simulink model "FOC_PMSM_FVSensorNew_testing"  (R2018b)
settings: Solver=ode45  StartTime=0  StopTime=0.2  FixedStep=1/fs/4  MaxStep=1/fs/2  RelTol=1e-7  EnableMultiTasking=on
InitFcn:
  | Motor_parameters_Lsrpm7fw
values from neighbouring files (symbols this model uses):
  fs = 20e3    (= 20000)    [Motor_parameters_Lsrpm7fw.m]
  Iphmax = I_rated*sqrt(2)*3    [Motor_parameters_Lsrpm7fw.m]
  J = 1*1e-3    (= 0.001)    [Motor_parameters_Lsrpm7fw.m]
  Ki1 = 2    [Motor_parameters_Lsrpm7fw.m]
  Ki2 = 6000    [Motor_parameters_Lsrpm7fw.m]
  Ki_pll = Bw^2*(1.1-0.334*zeta)^2*1/(2*k1)    (= 426432.888597)    [Motor_parameters_Lsrpm7fw.m]
  Kp1 = 0.05    [Motor_parameters_Lsrpm7fw.m]
  Kp2 = 6    [Motor_parameters_Lsrpm7fw.m]
  Kp_pll = Bw*(2.2*zeta-0.668*zeta^2)*1/(2*k1)    (= 13960.00992)    [Motor_parameters_Lsrpm7fw.m]
  Ld = 10e-3    (= 0.01)    [Motor_parameters_Lsrpm7fw.m]
  Lndd_ini = Lndmpm    (= 0.412)    [Motor_parameters_Lsrpm7fw.m]
  Lndmpm = 0.412    [Motor_parameters_Lsrpm7fw.m]
  Lq = 12.8e-3    (= 0.0128)    [Motor_parameters_Lsrpm7fw.m]
  Npp = 8/2    (= 4)    [Motor_parameters_Lsrpm7fw.m]
  Omegae_ini = 0    [Motor_parameters_Lsrpm7fw.m]
  Rs = 0.78    [Motor_parameters_Lsrpm7fw.m]
  Tl_const = Trat/nrat^2    (= 1.24081632653e-05)    [Motor_parameters_Lsrpm7fw.m]
  Trat = 38    [Motor_parameters_Lsrpm7fw.m]
  Vm = 70    [Motor_parameters_Lsrpm7fw.m]
  Vph = Vs*sqrt(2)    [Motor_parameters_Lsrpm7fw.m]
undefined symbols (not defined in the file or in its folder): DiscIntNeverNeededParam, plecs, sigbuilder_block
libraries: simulink x1
(part 2 of 2)

== system FOC_PMSM_FVSensorNew_testing/Rotor Pos. estimation/Cal. stator flux linkage/MinMax detection ==
  In : Inport
  Gain : Gain  Gain=1/2
  Max. Det : Subsystem
  Min. Det : Subsystem
  Mux6 : Mux  Inputs=3
  Scope5 : Scope
  Sum : Sum  Inputs=|++
  max.ou : Outport
  min.ou : Outport  Port=2
  average : Outport  Port=3
  wires:
  Gain/1 -> average/1
  Sum/1 -> Gain/1
  Max. Det/1(Max) -> max.ou/1, Mux6/1, Sum/1
  Min. Det/1(Min) -> min.ou/1, Mux6/3, Sum/2
  Mux6/1 -> Scope5/1
  In/1 -> Max. Det/1(In), Min. Det/1(In), Mux6/2

== system FOC_PMSM_FVSensorNew_testing/Rotor Pos. estimation/Cal. stator flux linkage1/MinMax detection ==
  In : Inport
  Gain : Gain  Gain=1/2
  Max. Det : Subsystem
  Min. Det : Subsystem
  Mux6 : Mux  Inputs=3
  Scope5 : Scope
  Sum : Sum  Inputs=|++
  max.ou : Outport
  min.ou : Outport  Port=2
  average : Outport  Port=3
  wires:
  Gain/1 -> average/1
  Sum/1 -> Gain/1
  Max. Det/1(Max) -> max.ou/1, Mux6/1, Sum/1
  Min. Det/1(Min) -> min.ou/1, Mux6/3, Sum/2
  Mux6/1 -> Scope5/1
  In/1 -> Max. Det/1(In), Min. Det/1(In), Mux6/2

== system FOC_PMSM_FVSensorNew_testing/Switch logic for sensorless vs sensor mode/Scope/ InputMux  ==
  In1 : Inport
  Convert1 : DataTypeConversion  SaturateOnIntegerOverflow=on  RndMeth=Zero
  Mux : Mux  Inputs=1
  Out : Outport
  wires:
  Convert1/1 -> Mux/1
  In1/1 -> Convert1/1
  Mux/1 -> Out/1

== system FOC_PMSM_FVSensorNew_testing/Switch logic for sensorless vs sensor mode/Scope1/ InputMux  ==
  In1 : Inport
  Convert1 : DataTypeConversion  SaturateOnIntegerOverflow=on  RndMeth=Zero
  Mux : Mux  Inputs=1
  Out : Outport
  wires:
  Mux/1 -> Out/1
  In1/1 -> Convert1/1
  Convert1/1 -> Mux/1

== system FOC_PMSM_FVSensorNew_testing/Rotor Pos. estimation/Cal. stator flux linkage/MinMax detection/Max. Det ==
  In : Inport
  Counter.1 : Subsystem
  Counter.2 : Subsystem
  Gain1 : Gain
  Gain2 : Gain  Gain=0.3
  Gain3 : Gain  Gain=0.6
  Mux2 : Mux
  Product : Product  RndMeth=Zero
  Relational Operator : RelationalOperator  RndMeth=Nearest
  Scope3 : Scope
  Unit Delay : UnitDelay  SampleTime=-1
  max.1 : Subsystem
  max.3 : Subsystem
  Max : Outport
  wires:
  Unit Delay/1 -> Relational Operator/2
  In/1 -> Unit Delay/1, max.1/1(In), Relational Operator/1, Mux2/1
  Relational Operator/1 -> max.1/Trigger, Counter.1/1(Sig.In), Counter.2/1(Sig.In), Gain1/1
  max.1/1(Out) -> max.3/1(In)
  Counter.1/1(En) -> Product/2, Gain3/1
  Mux2/1 -> Scope3/1
  Counter.2/1(En) -> Product/1, Gain2/1
  Product/1 -> max.3/Trigger
  Gain1/1 -> Mux2/2
  Gain2/1 -> Mux2/3
  Gain3/1 -> Mux2/4
  max.3/1(Out) -> Max/1

== system FOC_PMSM_FVSensorNew_testing/Rotor Pos. estimation/Cal. stator flux linkage/MinMax detection/Min. Det ==
  In : Inport
  Counter.1 : Subsystem
  Counter.2 : Subsystem
  Gain1 : Gain
  Gain2 : Gain  Gain=0.3
  Gain3 : Gain  Gain=0.6
  Mux2 : Mux
  Product : Product  RndMeth=Zero
  Relational Operator : RelationalOperator  Operator=<=  RndMeth=Nearest
  Scope3 : Scope
  Unit Delay : UnitDelay  SampleTime=-1
  max.1 : Subsystem
  max.3 : Subsystem
  Min : Outport
  wires:
  max.3/1(Out) -> Min/1
  Gain3/1 -> Mux2/4
  Gain2/1 -> Mux2/3
  Gain1/1 -> Mux2/2
  Product/1 -> max.3/Trigger
  Counter.2/1(En) -> Gain2/1, Product/1
  Mux2/1 -> Scope3/1
  Counter.1/1(En) -> Gain3/1, Product/2
  max.1/1(Out) -> max.3/1(In)
  Relational Operator/1 -> Gain1/1, Counter.2/1(Sig.In), Counter.1/1(Sig.In), max.1/Trigger
  In/1 -> Mux2/1, Relational Operator/1, max.1/1(In), Unit Delay/1
  Unit Delay/1 -> Relational Operator/2

== system FOC_PMSM_FVSensorNew_testing/Rotor Pos. estimation/Cal. stator flux linkage1/MinMax detection/Max. Det ==
  In : Inport
  Counter.1 : Subsystem
  Counter.2 : Subsystem
  Gain1 : Gain
  Gain2 : Gain  Gain=0.3
  Gain3 : Gain  Gain=0.6
  Mux2 : Mux
  Product : Product  RndMeth=Zero
  Relational Operator : RelationalOperator  RndMeth=Nearest
  Scope3 : Scope
  Unit Delay : UnitDelay  SampleTime=-1
  max.1 : Subsystem
  max.3 : Subsystem
  Max : Outport
  wires:
  Unit Delay/1 -> Relational Operator/2
  In/1 -> Unit Delay/1, max.1/1(In), Relational Operator/1, Mux2/1
  Relational Operator/1 -> max.1/Trigger, Counter.1/1(Sig.In), Counter.2/1(Sig.In), Gain1/1
  max.1/1(Out) -> max.3/1(In)
  Counter.1/1(En) -> Product/2, Gain3/1
  Mux2/1 -> Scope3/1
  Counter.2/1(En) -> Product/1, Gain2/1
  Product/1 -> max.3/Trigger
  Gain1/1 -> Mux2/2
  Gain2/1 -> Mux2/3
  Gain3/1 -> Mux2/4
  max.3/1(Out) -> Max/1

== system FOC_PMSM_FVSensorNew_testing/Rotor Pos. estimation/Cal. stator flux linkage1/MinMax detection/Min. Det ==
  In : Inport
  Counter.1 : Subsystem
  Counter.2 : Subsystem
  Gain1 : Gain
  Gain2 : Gain  Gain=0.3
  Gain3 : Gain  Gain=0.6
  Mux2 : Mux
  Product : Product  RndMeth=Zero
  Relational Operator : RelationalOperator  Operator=<=  RndMeth=Nearest
  Scope3 : Scope
  Unit Delay : UnitDelay  SampleTime=-1
  max.1 : Subsystem
  max.3 : Subsystem
  Min : Outport
  wires:
  max.3/1(Out) -> Min/1
  Gain3/1 -> Mux2/4
  Gain2/1 -> Mux2/3
  Gain1/1 -> Mux2/2
  Product/1 -> max.3/Trigger
  Counter.2/1(En) -> Gain2/1, Product/1
  Mux2/1 -> Scope3/1
  Counter.1/1(En) -> Gain3/1, Product/2
  max.1/1(Out) -> max.3/1(In)
  Relational Operator/1 -> Gain1/1, Counter.2/1(Sig.In), Counter.1/1(Sig.In), max.1/Trigger
  In/1 -> Mux2/1, Relational Operator/1, max.1/1(In), Unit Delay/1
  Unit Delay/1 -> Relational Operator/2

== system FOC_PMSM_FVSensorNew_testing/Rotor Pos. estimation/Cal. stator flux linkage/MinMax detection/Max. Det/Counter.1 ==
  Sig.In : Inport
  Constant4 : Constant  Value=10
  Constant5 : Constant
  Conter with enable : Subsystem
  Sum1 : Sum  Inputs=|-+
  En : Outport
  wires:
  Constant5/1 -> Sum1/2
  Sig.In/1 -> Sum1/1
  Conter with enable/1(Max. Reached?) -> En/1
  Sum1/1 -> Conter with enable/1(_|  |_)
  Constant4/1 -> Conter with enable/2(Max. Num)

== system FOC_PMSM_FVSensorNew_testing/Rotor Pos. estimation/Cal. stator flux linkage/MinMax detection/Max. Det/Counter.2 ==
  Sig.In : Inport
  Constant4 : Constant  Value=5
  Conter with enable : Subsystem
  Gain : Gain  Gain=2
  Gain1 : Gain  Gain=3
  Gain2 : Gain  Gain=4
  Mux1 : Mux
  Rising edge gen. : Subsystem
  SR Latch : Subsystem
  Scope2 : Scope
  En : Outport
  wires:
  Constant4/1 -> Conter with enable/2(Max. Num)
  Sig.In/1 -> Conter with enable/1(_|  |_), Rising edge gen./1(_|  |_), Gain2/1
  Conter with enable/1(Max. Reached?) -> SR Latch/2(S), Gain1/1
  SR Latch/1(Q) -> En/1, Mux1/1
  Mux1/1 -> Scope2/1
  Rising edge gen./1(Edge) -> SR Latch/1(R), Gain/1
  Gain/1 -> Mux1/2
  Gain1/1 -> Mux1/3
  Gain2/1 -> Mux1/4

== system FOC_PMSM_FVSensorNew_testing/Rotor Pos. estimation/Cal. stator flux linkage/MinMax detection/Max. Det/max.1 ==
  In : Inport
  Trigger : TriggerPort  TriggerType=falling  VariantControl=(inherit)
  Out : Outport
  wires:
  In/1 -> Out/1

== system FOC_PMSM_FVSensorNew_testing/Rotor Pos. estimation/Cal. stator flux linkage/MinMax detection/Max. Det/max.3 ==
  In : Inport
  Trigger : TriggerPort  VariantControl=(inherit)
  Out : Outport
  wires:
  In/1 -> Out/1

== system FOC_PMSM_FVSensorNew_testing/Rotor Pos. estimation/Cal. stator flux linkage/MinMax detection/Min. Det/Counter.1 ==
  Sig.In : Inport
  Constant4 : Constant  Value=10
  Constant5 : Constant
  Conter with enable : Subsystem
  Sum1 : Sum  Inputs=|-+
  En : Outport
  wires:
  Constant4/1 -> Conter with enable/2(Max. Num)
  Sum1/1 -> Conter with enable/1(_|  |_)
  Conter with enable/1(Max. Reached?) -> En/1
  Sig.In/1 -> Sum1/1
  Constant5/1 -> Sum1/2

== system FOC_PMSM_FVSensorNew_testing/Rotor Pos. estimation/Cal. stator flux linkage/MinMax detection/Min. Det/Counter.2 ==
  Sig.In : Inport
  Constant4 : Constant  Value=5
  Conter with enable : Subsystem
  Gain : Gain  Gain=2
  Gain1 : Gain  Gain=3
  Gain2 : Gain  Gain=4
  Mux1 : Mux
  Rising edge gen. : Subsystem
  SR Latch : Subsystem
  Scope2 : Scope
  En : Outport
  wires:
  Gain2/1 -> Mux1/4
  Gain1/1 -> Mux1/3
  Gain/1 -> Mux1/2
  Rising edge gen./1(Edge) -> Gain/1, SR Latch/1(R)
  Mux1/1 -> Scope2/1
  SR Latch/1(Q) -> Mux1/1, En/1
  Conter with enable/1(Max. Reached?) -> Gain1/1, SR Latch/2(S)
  Sig.In/1 -> Gain2/1, Rising edge gen./1(_|  |_), Conter with enable/1(_|  |_)
  Constant4/1 -> Conter with enable/2(Max. Num)

== system FOC_PMSM_FVSensorNew_testing/Rotor Pos. estimation/Cal. stator flux linkage/MinMax detection/Min. Det/max.1 ==
  In : Inport
  Trigger : TriggerPort  TriggerType=falling  VariantControl=(inherit)
  Out : Outport
  wires:
  In/1 -> Out/1

== system FOC_PMSM_FVSensorNew_testing/Rotor Pos. estimation/Cal. stator flux linkage/MinMax detection/Min. Det/max.3 ==
  In : Inport
  Trigger : TriggerPort  VariantControl=(inherit)
  Out : Outport
  wires:
  In/1 -> Out/1

== system FOC_PMSM_FVSensorNew_testing/Rotor Pos. estimation/Cal. stator flux linkage1/MinMax detection/Max. Det/Counter.1 ==
  Sig.In : Inport
  Constant4 : Constant  Value=10
  Constant5 : Constant
  Conter with enable : Subsystem
  Sum1 : Sum  Inputs=|-+
  En : Outport
  wires:
  Constant5/1 -> Sum1/2
  Sig.In/1 -> Sum1/1
  Conter with enable/1(Max. Reached?) -> En/1
  Sum1/1 -> Conter with enable/1(_|  |_)
  Constant4/1 -> Conter with enable/2(Max. Num)

== system FOC_PMSM_FVSensorNew_testing/Rotor Pos. estimation/Cal. stator flux linkage1/MinMax detection/Max. Det/Counter.2 ==
  Sig.In : Inport
  Constant4 : Constant  Value=5
  Conter with enable : Subsystem
  Gain : Gain  Gain=2
  Gain1 : Gain  Gain=3
  Gain2 : Gain  Gain=4
  Mux1 : Mux
  Rising edge gen. : Subsystem
  SR Latch : Subsystem
  Scope2 : Scope
  En : Outport
  wires:
  Constant4/1 -> Conter with enable/2(Max. Num)
  Sig.In/1 -> Conter with enable/1(_|  |_), Rising edge gen./1(_|  |_), Gain2/1
  Conter with enable/1(Max. Reached?) -> SR Latch/2(S), Gain1/1
  SR Latch/1(Q) -> En/1, Mux1/1
  Mux1/1 -> Scope2/1
  Rising edge gen./1(Edge) -> SR Latch/1(R), Gain/1
  Gain/1 -> Mux1/2
  Gain1/1 -> Mux1/3
  Gain2/1 -> Mux1/4

== system FOC_PMSM_FVSensorNew_testing/Rotor Pos. estimation/Cal. stator flux linkage1/MinMax detection/Max. Det/max.1 ==
  In : Inport
  Trigger : TriggerPort  TriggerType=falling  VariantControl=(inherit)
  Out : Outport
  wires:
  In/1 -> Out/1

== system FOC_PMSM_FVSensorNew_testing/Rotor Pos. estimation/Cal. stator flux linkage1/MinMax detection/Max. Det/max.3 ==
  In : Inport
  Trigger : TriggerPort  VariantControl=(inherit)
  Out : Outport
  wires:
  In/1 -> Out/1

== system FOC_PMSM_FVSensorNew_testing/Rotor Pos. estimation/Cal. stator flux linkage1/MinMax detection/Min. Det/Counter.1 ==
  Sig.In : Inport
  Constant4 : Constant  Value=10
  Constant5 : Constant
  Conter with enable : Subsystem
  Sum1 : Sum  Inputs=|-+
  En : Outport
  wires:
  Constant4/1 -> Conter with enable/2(Max. Num)
  Sum1/1 -> Conter with enable/1(_|  |_)
  Conter with enable/1(Max. Reached?) -> En/1
  Sig.In/1 -> Sum1/1
  Constant5/1 -> Sum1/2

== system FOC_PMSM_FVSensorNew_testing/Rotor Pos. estimation/Cal. stator flux linkage1/MinMax detection/Min. Det/Counter.2 ==
  Sig.In : Inport
  Constant4 : Constant  Value=5
  Conter with enable : Subsystem
  Gain : Gain  Gain=2
  Gain1 : Gain  Gain=3
  Gain2 : Gain  Gain=4
  Mux1 : Mux
  Rising edge gen. : Subsystem
  SR Latch : Subsystem
  Scope2 : Scope
  En : Outport
  wires:
  Gain2/1 -> Mux1/4
  Gain1/1 -> Mux1/3
  Gain/1 -> Mux1/2
  Rising edge gen./1(Edge) -> Gain/1, SR Latch/1(R)
  Mux1/1 -> Scope2/1
  SR Latch/1(Q) -> Mux1/1, En/1
  Conter with enable/1(Max. Reached?) -> Gain1/1, SR Latch/2(S)
  Sig.In/1 -> Gain2/1, Rising edge gen./1(_|  |_), Conter with enable/1(_|  |_)
  Constant4/1 -> Conter with enable/2(Max. Num)

== system FOC_PMSM_FVSensorNew_testing/Rotor Pos. estimation/Cal. stator flux linkage1/MinMax detection/Min. Det/max.1 ==
  In : Inport
  Trigger : TriggerPort  TriggerType=falling  VariantControl=(inherit)
  Out : Outport
  wires:
  In/1 -> Out/1

== system FOC_PMSM_FVSensorNew_testing/Rotor Pos. estimation/Cal. stator flux linkage1/MinMax detection/Min. Det/max.3 ==
  In : Inport
  Trigger : TriggerPort  VariantControl=(inherit)
  Out : Outport
  wires:
  In/1 -> Out/1

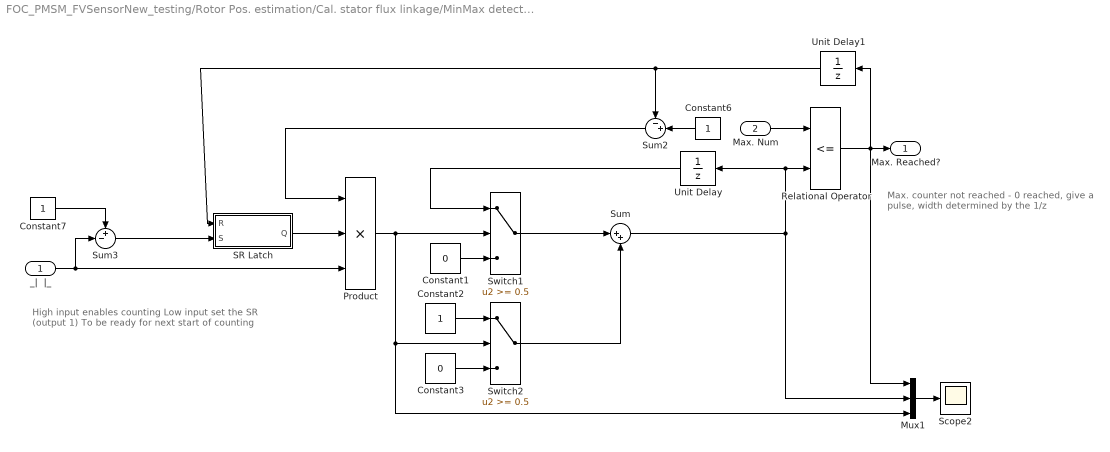
== system FOC_PMSM_FVSensorNew_testing/Rotor Pos. estimation/Cal. stator flux linkage/MinMax detection/Max. Det/Counter.1/Conter with enable ==
  note: High input enables counting
      | Low input set the SR (output 1)
      | To be ready for next start of
      | counting
  note: Max. counter not reached - 0
      | reached, give a pulse, width
      | determined by the 1/z
  _|  |_ : Inport
  Max. Num : Inport  Port=2
  Constant1 : Constant  Value=0
  Constant2 : Constant
  Constant3 : Constant  Value=0
  Constant6 : Constant
  Constant7 : Constant
  Mux1 : Mux  Inputs=3
  Product : Product  Inputs=3  RndMeth=Zero
  Relational Operator : RelationalOperator  Operator=<=  RndMeth=Nearest
  SR Latch : Subsystem
  Scope2 : Scope
  Sum : Sum  Inputs=|++
  Sum2 : Sum  Inputs=-+|
  Sum3 : Sum  Inputs=+-|
  Switch1 : Switch  Threshold=0.5
  Switch2 : Switch  Threshold=0.5
  Unit Delay : UnitDelay  SampleTime=-1
  Unit Delay1 : UnitDelay  SampleTime=-1
  Max. Reached? : Outport
  wires:
  Constant1/1 -> Switch1/3
  Constant2/1 -> Switch2/1
  Constant3/1 -> Switch2/3
  Switch1/1 -> Sum/1
  Switch2/1 -> Sum/2
  Sum/1 -> Unit Delay/1, Relational Operator/2, Mux1/2
  Unit Delay/1 -> Switch1/1
  Max. Num/1 -> Relational Operator/1
  Relational Operator/1 -> Mux1/1, Unit Delay1/1, Max. Reached?/1
  Mux1/1 -> Scope2/1
  Sum2/1 -> Product/1
  Product/1 -> Switch1/2, Switch2/2, Mux1/3
  _|  |_/1 -> Sum3/2, Product/3
  SR Latch/1(Q) -> Product/2
  Sum3/1 -> SR Latch/2(S)
  Constant7/1 -> Sum3/1
  Constant6/1 -> Sum2/2
  Unit Delay1/1 -> Sum2/1, SR Latch/1(R)

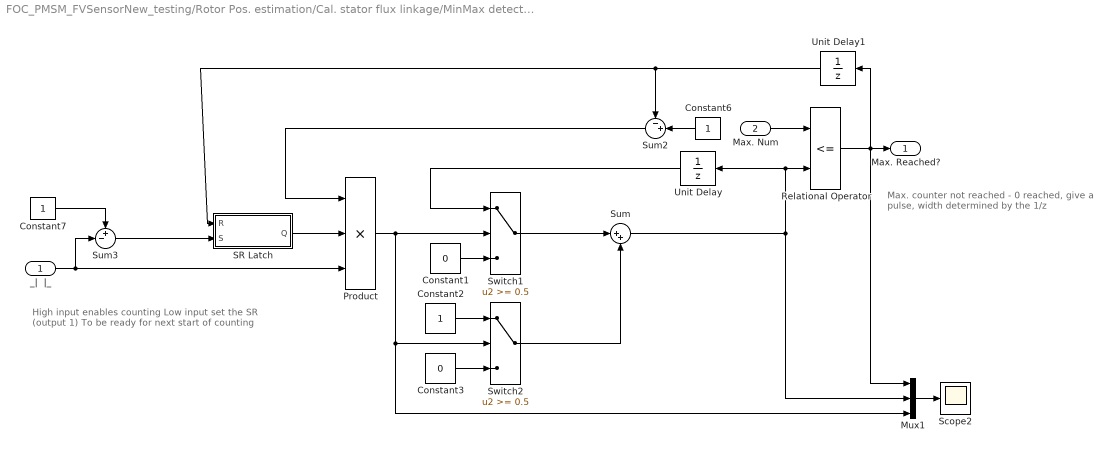
== system FOC_PMSM_FVSensorNew_testing/Rotor Pos. estimation/Cal. stator flux linkage/MinMax detection/Max. Det/Counter.2/Conter with enable ==
  note: Max. counter not reached - 0
      | reached, give a pulse, width
      | determined by the 1/z
  note: High input enables counting
      | Low input set the SR (output 1)
      | To be ready for next start of
      | counting
  _|  |_ : Inport
  Max. Num : Inport  Port=2
  Constant1 : Constant  Value=0
  Constant2 : Constant
  Constant3 : Constant  Value=0
  Constant6 : Constant
  Constant7 : Constant
  Mux1 : Mux  Inputs=3
  Product : Product  Inputs=3  RndMeth=Zero
  Relational Operator : RelationalOperator  Operator=<=  RndMeth=Nearest
  SR Latch : Subsystem
  Scope2 : Scope
  Sum : Sum  Inputs=|++
  Sum2 : Sum  Inputs=-+|
  Sum3 : Sum  Inputs=+-|
  Switch1 : Switch  Threshold=0.5
  Switch2 : Switch  Threshold=0.5
  Unit Delay : UnitDelay  SampleTime=-1
  Unit Delay1 : UnitDelay  SampleTime=-1
  Max. Reached? : Outport
  wires:
  Unit Delay1/1 -> SR Latch/1(R), Sum2/1
  Constant6/1 -> Sum2/2
  Constant7/1 -> Sum3/1
  Sum3/1 -> SR Latch/2(S)
  SR Latch/1(Q) -> Product/2
  _|  |_/1 -> Product/3, Sum3/2
  Product/1 -> Mux1/3, Switch2/2, Switch1/2
  Sum2/1 -> Product/1
  Mux1/1 -> Scope2/1
  Relational Operator/1 -> Max. Reached?/1, Unit Delay1/1, Mux1/1
  Max. Num/1 -> Relational Operator/1
  Unit Delay/1 -> Switch1/1
  Sum/1 -> Mux1/2, Relational Operator/2, Unit Delay/1
  Switch2/1 -> Sum/2
  Switch1/1 -> Sum/1
  Constant3/1 -> Switch2/3
  Constant2/1 -> Switch2/1
  Constant1/1 -> Switch1/3

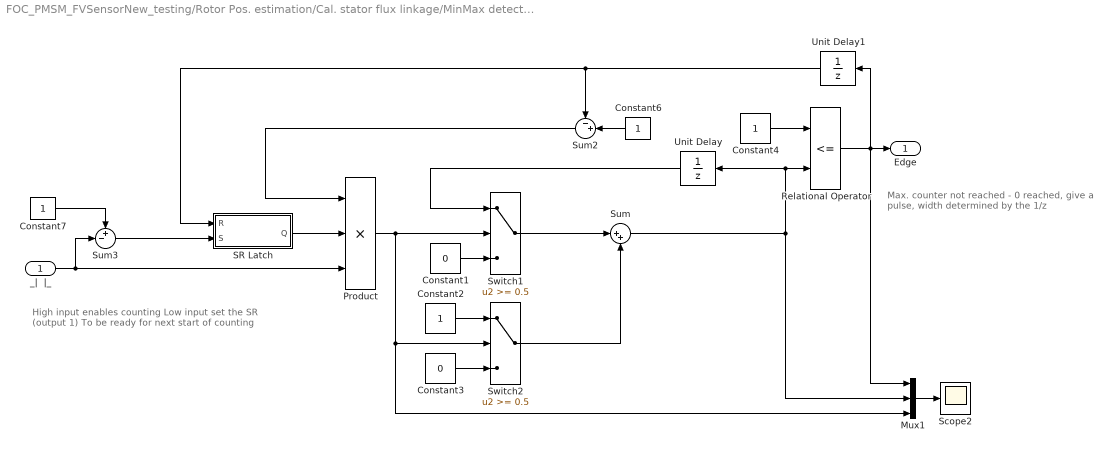
== system FOC_PMSM_FVSensorNew_testing/Rotor Pos. estimation/Cal. stator flux linkage/MinMax detection/Max. Det/Counter.2/Rising edge gen. ==
  note: High input enables counting
      | Low input set the SR (output 1)
      | To be ready for next start of
      | counting
  note: Max. counter not reached - 0
      | reached, give a pulse, width
      | determined by the 1/z
  _|  |_ : Inport
  Constant1 : Constant  Value=0
  Constant{2,4,6..7} (4 alike) : Constant
  Constant3 : Constant  Value=0
  Mux1 : Mux  Inputs=3
  Product : Product  Inputs=3  RndMeth=Zero
  Relational Operator : RelationalOperator  Operator=<=  RndMeth=Nearest
  SR Latch : Subsystem
  Scope2 : Scope
  Sum : Sum  Inputs=|++
  Sum2 : Sum  Inputs=-+|
  Sum3 : Sum  Inputs=+-|
  Switch1 : Switch  Threshold=0.5
  Switch2 : Switch  Threshold=0.5
  Unit Delay : UnitDelay  SampleTime=-1
  Unit Delay1 : UnitDelay  SampleTime=-1
  Edge : Outport
  wires:
  Constant1/1 -> Switch1/3
  Constant2/1 -> Switch2/1
  Constant3/1 -> Switch2/3
  Switch1/1 -> Sum/1
  Switch2/1 -> Sum/2
  Sum/1 -> Unit Delay/1, Relational Operator/2, Mux1/2
  Unit Delay/1 -> Switch1/1
  Constant4/1 -> Relational Operator/1
  Relational Operator/1 -> Mux1/1, Unit Delay1/1, Edge/1
  Mux1/1 -> Scope2/1
  Sum2/1 -> Product/1
  Product/1 -> Switch1/2, Switch2/2, Mux1/3
  _|  |_/1 -> Sum3/2, Product/3
  SR Latch/1(Q) -> Product/2
  Sum3/1 -> SR Latch/2(S)
  Constant7/1 -> Sum3/1
  Constant6/1 -> Sum2/2
  Unit Delay1/1 -> Sum2/1, SR Latch/1(R)

== system FOC_PMSM_FVSensorNew_testing/Rotor Pos. estimation/Cal. stator flux linkage/MinMax detection/Max. Det/Counter.2/SR Latch ==
  R : Inport
  S : Inport  Port=2
  Constant2 : Constant
  Constant4 : Constant  Value=0
  Constant5 : Constant  Value=0
  Multiport Switch : MultiPortSwitch  Inputs=4
  Mux1 : Mux  Inputs=2
  Selcect : Fcn  Expr=(1-u(1))*(1-u(2))+2*(1-u(1))*u(2)+3*u(1)*(1-u(2))+4*u(1)*u(2)
  Unit Delay2 : UnitDelay  SampleTime=-1
  Q : Outport
  wires:
  S/1 -> Mux1/2
  R/1 -> Mux1/1
  Constant5/1 -> Multiport Switch/5
  Constant4/1 -> Multiport Switch/4
  Constant2/1 -> Multiport Switch/3
  Unit Delay2/1 -> Multiport Switch/2
  Mux1/1 -> Selcect/1
  Selcect/1 -> Multiport Switch/1
  Multiport Switch/1 -> Unit Delay2/1, Q/1

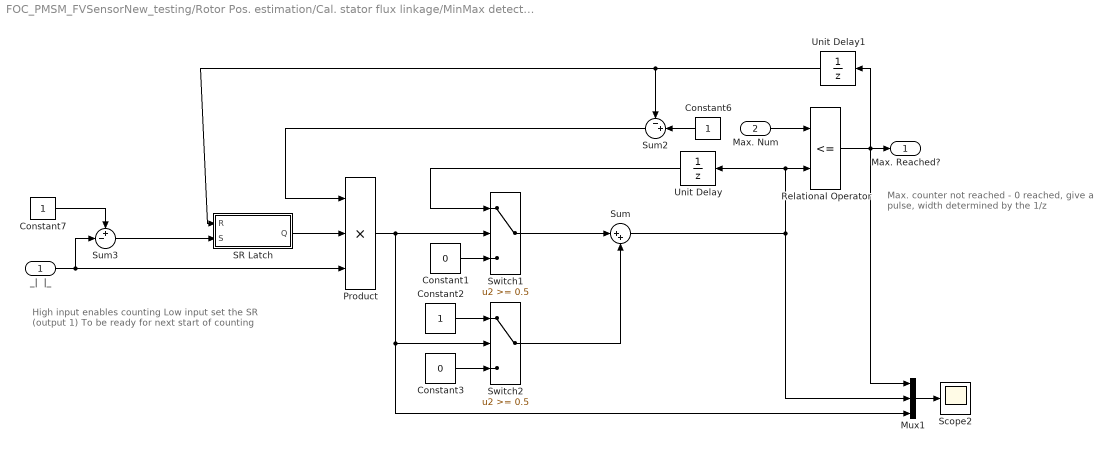
== system FOC_PMSM_FVSensorNew_testing/Rotor Pos. estimation/Cal. stator flux linkage/MinMax detection/Min. Det/Counter.1/Conter with enable ==
  note: Max. counter not reached - 0
      | reached, give a pulse, width
      | determined by the 1/z
  note: High input enables counting
      | Low input set the SR (output 1)
      | To be ready for next start of
      | counting
  _|  |_ : Inport
  Max. Num : Inport  Port=2
  Constant1 : Constant  Value=0
  Constant2 : Constant
  Constant3 : Constant  Value=0
  Constant6 : Constant
  Constant7 : Constant
  Mux1 : Mux  Inputs=3
  Product : Product  Inputs=3  RndMeth=Zero
  Relational Operator : RelationalOperator  Operator=<=  RndMeth=Nearest
  SR Latch : Subsystem
  Scope2 : Scope
  Sum : Sum  Inputs=|++
  Sum2 : Sum  Inputs=-+|
  Sum3 : Sum  Inputs=+-|
  Switch1 : Switch  Threshold=0.5
  Switch2 : Switch  Threshold=0.5
  Unit Delay : UnitDelay  SampleTime=-1
  Unit Delay1 : UnitDelay  SampleTime=-1
  Max. Reached? : Outport
  wires:
  Unit Delay1/1 -> SR Latch/1(R), Sum2/1
  Constant6/1 -> Sum2/2
  Constant7/1 -> Sum3/1
  Sum3/1 -> SR Latch/2(S)
  SR Latch/1(Q) -> Product/2
  _|  |_/1 -> Product/3, Sum3/2
  Product/1 -> Mux1/3, Switch2/2, Switch1/2
  Sum2/1 -> Product/1
  Mux1/1 -> Scope2/1
  Relational Operator/1 -> Max. Reached?/1, Unit Delay1/1, Mux1/1
  Max. Num/1 -> Relational Operator/1
  Unit Delay/1 -> Switch1/1
  Sum/1 -> Mux1/2, Relational Operator/2, Unit Delay/1
  Switch2/1 -> Sum/2
  Switch1/1 -> Sum/1
  Constant3/1 -> Switch2/3
  Constant2/1 -> Switch2/1
  Constant1/1 -> Switch1/3

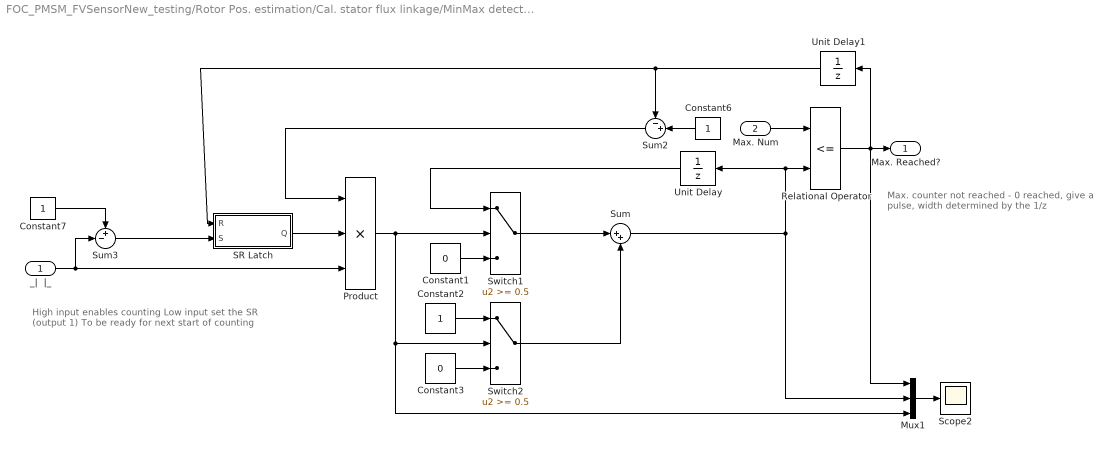
== system FOC_PMSM_FVSensorNew_testing/Rotor Pos. estimation/Cal. stator flux linkage/MinMax detection/Min. Det/Counter.2/Conter with enable ==
  note: High input enables counting
      | Low input set the SR (output 1)
      | To be ready for next start of
      | counting
  note: Max. counter not reached - 0
      | reached, give a pulse, width
      | determined by the 1/z
  _|  |_ : Inport
  Max. Num : Inport  Port=2
  Constant1 : Constant  Value=0
  Constant2 : Constant
  Constant3 : Constant  Value=0
  Constant6 : Constant
  Constant7 : Constant
  Mux1 : Mux  Inputs=3
  Product : Product  Inputs=3  RndMeth=Zero
  Relational Operator : RelationalOperator  Operator=<=  RndMeth=Nearest
  SR Latch : Subsystem
  Scope2 : Scope
  Sum : Sum  Inputs=|++
  Sum2 : Sum  Inputs=-+|
  Sum3 : Sum  Inputs=+-|
  Switch1 : Switch  Threshold=0.5
  Switch2 : Switch  Threshold=0.5
  Unit Delay : UnitDelay  SampleTime=-1
  Unit Delay1 : UnitDelay  SampleTime=-1
  Max. Reached? : Outport
  wires:
  Constant1/1 -> Switch1/3
  Constant2/1 -> Switch2/1
  Constant3/1 -> Switch2/3
  Switch1/1 -> Sum/1
  Switch2/1 -> Sum/2
  Sum/1 -> Unit Delay/1, Relational Operator/2, Mux1/2
  Unit Delay/1 -> Switch1/1
  Max. Num/1 -> Relational Operator/1
  Relational Operator/1 -> Mux1/1, Unit Delay1/1, Max. Reached?/1
  Mux1/1 -> Scope2/1
  Sum2/1 -> Product/1
  Product/1 -> Switch1/2, Switch2/2, Mux1/3
  _|  |_/1 -> Sum3/2, Product/3
  SR Latch/1(Q) -> Product/2
  Sum3/1 -> SR Latch/2(S)
  Constant7/1 -> Sum3/1
  Constant6/1 -> Sum2/2
  Unit Delay1/1 -> Sum2/1, SR Latch/1(R)

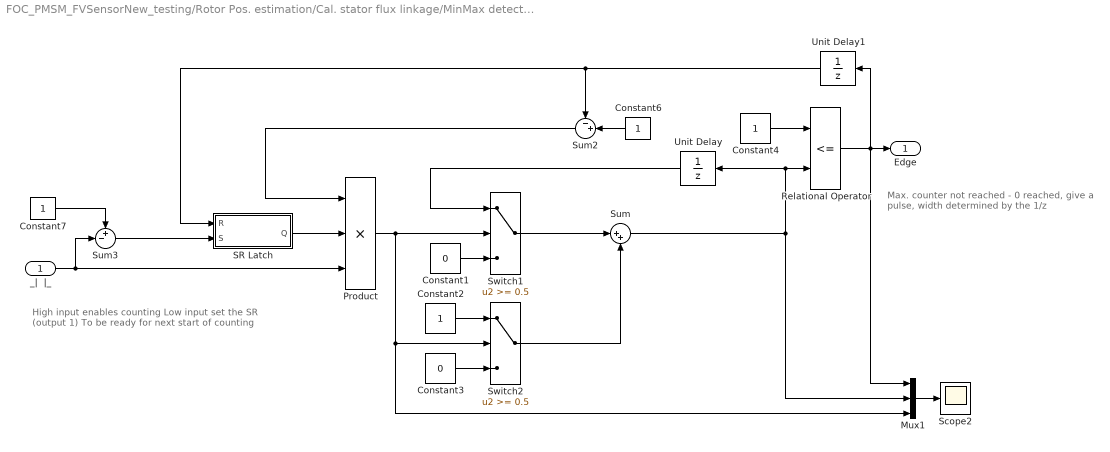
== system FOC_PMSM_FVSensorNew_testing/Rotor Pos. estimation/Cal. stator flux linkage/MinMax detection/Min. Det/Counter.2/Rising edge gen. ==
  note: Max. counter not reached - 0
      | reached, give a pulse, width
      | determined by the 1/z
  note: High input enables counting
      | Low input set the SR (output 1)
      | To be ready for next start of
      | counting
  _|  |_ : Inport
  Constant1 : Constant  Value=0
  Constant{2,4,6..7} (4 alike) : Constant
  Constant3 : Constant  Value=0
  Mux1 : Mux  Inputs=3
  Product : Product  Inputs=3  RndMeth=Zero
  Relational Operator : RelationalOperator  Operator=<=  RndMeth=Nearest
  SR Latch : Subsystem
  Scope2 : Scope
  Sum : Sum  Inputs=|++
  Sum2 : Sum  Inputs=-+|
  Sum3 : Sum  Inputs=+-|
  Switch1 : Switch  Threshold=0.5
  Switch2 : Switch  Threshold=0.5
  Unit Delay : UnitDelay  SampleTime=-1
  Unit Delay1 : UnitDelay  SampleTime=-1
  Edge : Outport
  wires:
  Unit Delay1/1 -> SR Latch/1(R), Sum2/1
  Constant6/1 -> Sum2/2
  Constant7/1 -> Sum3/1
  Sum3/1 -> SR Latch/2(S)
  SR Latch/1(Q) -> Product/2
  _|  |_/1 -> Product/3, Sum3/2
  Product/1 -> Mux1/3, Switch2/2, Switch1/2
  Sum2/1 -> Product/1
  Mux1/1 -> Scope2/1
  Relational Operator/1 -> Edge/1, Unit Delay1/1, Mux1/1
  Constant4/1 -> Relational Operator/1
  Unit Delay/1 -> Switch1/1
  Sum/1 -> Mux1/2, Relational Operator/2, Unit Delay/1
  Switch2/1 -> Sum/2
  Switch1/1 -> Sum/1
  Constant3/1 -> Switch2/3
  Constant2/1 -> Switch2/1
  Constant1/1 -> Switch1/3

== system FOC_PMSM_FVSensorNew_testing/Rotor Pos. estimation/Cal. stator flux linkage/MinMax detection/Min. Det/Counter.2/SR Latch ==
  R : Inport
  S : Inport  Port=2
  Constant2 : Constant
  Constant4 : Constant  Value=0
  Constant5 : Constant  Value=0
  Multiport Switch : MultiPortSwitch  Inputs=4
  Mux1 : Mux  Inputs=2
  Selcect : Fcn  Expr=(1-u(1))*(1-u(2))+2*(1-u(1))*u(2)+3*u(1)*(1-u(2))+4*u(1)*u(2)
  Unit Delay2 : UnitDelay  SampleTime=-1
  Q : Outport
  wires:
  Multiport Switch/1 -> Q/1, Unit Delay2/1
  Selcect/1 -> Multiport Switch/1
  Mux1/1 -> Selcect/1
  Unit Delay2/1 -> Multiport Switch/2
  Constant2/1 -> Multiport Switch/3
  Constant4/1 -> Multiport Switch/4
  Constant5/1 -> Multiport Switch/5
  R/1 -> Mux1/1
  S/1 -> Mux1/2

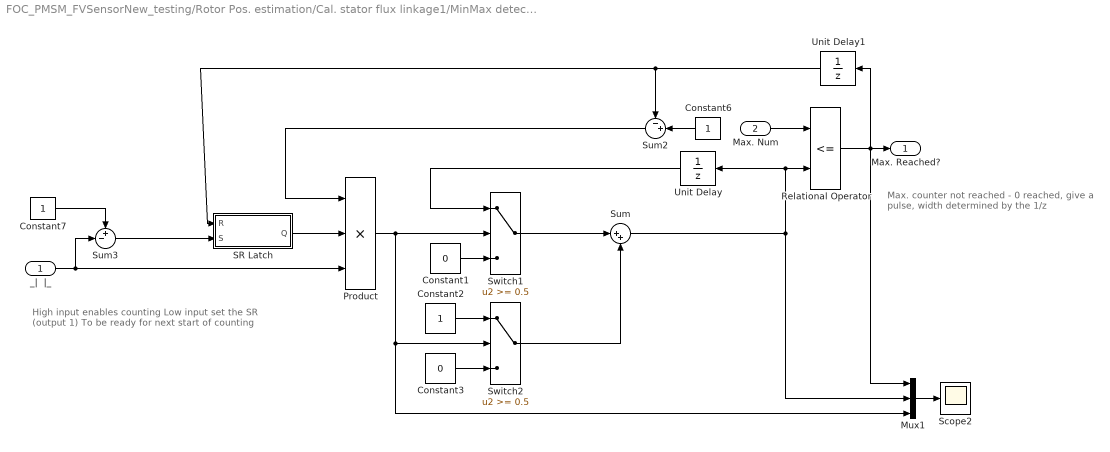
== system FOC_PMSM_FVSensorNew_testing/Rotor Pos. estimation/Cal. stator flux linkage1/MinMax detection/Max. Det/Counter.1/Conter with enable ==
  note: High input enables counting
      | Low input set the SR (output 1)
      | To be ready for next start of
      | counting
  note: Max. counter not reached - 0
      | reached, give a pulse, width
      | determined by the 1/z
  _|  |_ : Inport
  Max. Num : Inport  Port=2
  Constant1 : Constant  Value=0
  Constant2 : Constant
  Constant3 : Constant  Value=0
  Constant6 : Constant
  Constant7 : Constant
  Mux1 : Mux  Inputs=3
  Product : Product  Inputs=3  RndMeth=Zero
  Relational Operator : RelationalOperator  Operator=<=  RndMeth=Nearest
  SR Latch : Subsystem
  Scope2 : Scope
  Sum : Sum  Inputs=|++
  Sum2 : Sum  Inputs=-+|
  Sum3 : Sum  Inputs=+-|
  Switch1 : Switch  Threshold=0.5
  Switch2 : Switch  Threshold=0.5
  Unit Delay : UnitDelay  SampleTime=-1
  Unit Delay1 : UnitDelay  SampleTime=-1
  Max. Reached? : Outport
  wires:
  Constant1/1 -> Switch1/3
  Constant2/1 -> Switch2/1
  Constant3/1 -> Switch2/3
  Switch1/1 -> Sum/1
  Switch2/1 -> Sum/2
  Sum/1 -> Unit Delay/1, Relational Operator/2, Mux1/2
  Unit Delay/1 -> Switch1/1
  Max. Num/1 -> Relational Operator/1
  Relational Operator/1 -> Mux1/1, Unit Delay1/1, Max. Reached?/1
  Mux1/1 -> Scope2/1
  Sum2/1 -> Product/1
  Product/1 -> Switch1/2, Switch2/2, Mux1/3
  _|  |_/1 -> Sum3/2, Product/3
  SR Latch/1(Q) -> Product/2
  Sum3/1 -> SR Latch/2(S)
  Constant7/1 -> Sum3/1
  Constant6/1 -> Sum2/2
  Unit Delay1/1 -> Sum2/1, SR Latch/1(R)

== system FOC_PMSM_FVSensorNew_testing/Rotor Pos. estimation/Cal. stator flux linkage1/MinMax detection/Max. Det/Counter.2/Conter with enable ==
  note: Max. counter not reached - 0
      | reached, give a pulse, width
      | determined by the 1/z
  note: High input enables counting
      | Low input set the SR (output 1)
      | To be ready for next start of
      | counting
  _|  |_ : Inport
  Max. Num : Inport  Port=2
  Constant1 : Constant  Value=0
  Constant2 : Constant
  Constant3 : Constant  Value=0
  Constant6 : Constant
  Constant7 : Constant
  Mux1 : Mux  Inputs=3
  Product : Product  Inputs=3  RndMeth=Zero
  Relational Operator : RelationalOperator  Operator=<=  RndMeth=Nearest
  SR Latch : Subsystem
  Scope2 : Scope
  Sum : Sum  Inputs=|++
  Sum2 : Sum  Inputs=-+|
  Sum3 : Sum  Inputs=+-|
  Switch1 : Switch  Threshold=0.5
  Switch2 : Switch  Threshold=0.5
  Unit Delay : UnitDelay  SampleTime=-1
  Unit Delay1 : UnitDelay  SampleTime=-1
  Max. Reached? : Outport
  wires:
  Unit Delay1/1 -> SR Latch/1(R), Sum2/1
  Constant6/1 -> Sum2/2
  Constant7/1 -> Sum3/1
  Sum3/1 -> SR Latch/2(S)
  SR Latch/1(Q) -> Product/2
  _|  |_/1 -> Product/3, Sum3/2
  Product/1 -> Mux1/3, Switch2/2, Switch1/2
  Sum2/1 -> Product/1
  Mux1/1 -> Scope2/1
  Relational Operator/1 -> Max. Reached?/1, Unit Delay1/1, Mux1/1
  Max. Num/1 -> Relational Operator/1
  Unit Delay/1 -> Switch1/1
  Sum/1 -> Mux1/2, Relational Operator/2, Unit Delay/1
  Switch2/1 -> Sum/2
  Switch1/1 -> Sum/1
  Constant3/1 -> Switch2/3
  Constant2/1 -> Switch2/1
  Constant1/1 -> Switch1/3

== system FOC_PMSM_FVSensorNew_testing/Rotor Pos. estimation/Cal. stator flux linkage1/MinMax detection/Max. Det/Counter.2/Rising edge gen. ==
  note: High input enables counting
      | Low input set the SR (output 1)
      | To be ready for next start of
      | counting
  note: Max. counter not reached - 0
      | reached, give a pulse, width
      | determined by the 1/z
  _|  |_ : Inport
  Constant1 : Constant  Value=0
  Constant{2,4,6..7} (4 alike) : Constant
  Constant3 : Constant  Value=0
  Mux1 : Mux  Inputs=3
  Product : Product  Inputs=3  RndMeth=Zero
  Relational Operator : RelationalOperator  Operator=<=  RndMeth=Nearest
  SR Latch : Subsystem
  Scope2 : Scope
  Sum : Sum  Inputs=|++
  Sum2 : Sum  Inputs=-+|
  Sum3 : Sum  Inputs=+-|
  Switch1 : Switch  Threshold=0.5
  Switch2 : Switch  Threshold=0.5
  Unit Delay : UnitDelay  SampleTime=-1
  Unit Delay1 : UnitDelay  SampleTime=-1
  Edge : Outport
  wires:
  Constant1/1 -> Switch1/3
  Constant2/1 -> Switch2/1
  Constant3/1 -> Switch2/3
  Switch1/1 -> Sum/1
  Switch2/1 -> Sum/2
  Sum/1 -> Unit Delay/1, Relational Operator/2, Mux1/2
  Unit Delay/1 -> Switch1/1
  Constant4/1 -> Relational Operator/1
  Relational Operator/1 -> Mux1/1, Unit Delay1/1, Edge/1
  Mux1/1 -> Scope2/1
  Sum2/1 -> Product/1
  Product/1 -> Switch1/2, Switch2/2, Mux1/3
  _|  |_/1 -> Sum3/2, Product/3
  SR Latch/1(Q) -> Product/2
  Sum3/1 -> SR Latch/2(S)
  Constant7/1 -> Sum3/1
  Constant6/1 -> Sum2/2
  Unit Delay1/1 -> Sum2/1, SR Latch/1(R)

== system FOC_PMSM_FVSensorNew_testing/Rotor Pos. estimation/Cal. stator flux linkage1/MinMax detection/Max. Det/Counter.2/SR Latch ==
  R : Inport
  S : Inport  Port=2
  Constant2 : Constant
  Constant4 : Constant  Value=0
  Constant5 : Constant  Value=0
  Multiport Switch : MultiPortSwitch  Inputs=4
  Mux1 : Mux  Inputs=2
  Selcect : Fcn  Expr=(1-u(1))*(1-u(2))+2*(1-u(1))*u(2)+3*u(1)*(1-u(2))+4*u(1)*u(2)
  Unit Delay2 : UnitDelay  SampleTime=-1
  Q : Outport
  wires:
  S/1 -> Mux1/2
  R/1 -> Mux1/1
  Constant5/1 -> Multiport Switch/5
  Constant4/1 -> Multiport Switch/4
  Constant2/1 -> Multiport Switch/3
  Unit Delay2/1 -> Multiport Switch/2
  Mux1/1 -> Selcect/1
  Selcect/1 -> Multiport Switch/1
  Multiport Switch/1 -> Unit Delay2/1, Q/1

== system FOC_PMSM_FVSensorNew_testing/Rotor Pos. estimation/Cal. stator flux linkage1/MinMax detection/Min. Det/Counter.1/Conter with enable ==
  note: Max. counter not reached - 0
      | reached, give a pulse, width
      | determined by the 1/z
  note: High input enables counting
      | Low input set the SR (output 1)
      | To be ready for next start of
      | counting
  _|  |_ : Inport
  Max. Num : Inport  Port=2
  Constant1 : Constant  Value=0
  Constant2 : Constant
  Constant3 : Constant  Value=0
  Constant6 : Constant
  Constant7 : Constant
  Mux1 : Mux  Inputs=3
  Product : Product  Inputs=3  RndMeth=Zero
  Relational Operator : RelationalOperator  Operator=<=  RndMeth=Nearest
  SR Latch : Subsystem
  Scope2 : Scope
  Sum : Sum  Inputs=|++
  Sum2 : Sum  Inputs=-+|
  Sum3 : Sum  Inputs=+-|
  Switch1 : Switch  Threshold=0.5
  Switch2 : Switch  Threshold=0.5
  Unit Delay : UnitDelay  SampleTime=-1
  Unit Delay1 : UnitDelay  SampleTime=-1
  Max. Reached? : Outport
  wires:
  Unit Delay1/1 -> SR Latch/1(R), Sum2/1
  Constant6/1 -> Sum2/2
  Constant7/1 -> Sum3/1
  Sum3/1 -> SR Latch/2(S)
  SR Latch/1(Q) -> Product/2
  _|  |_/1 -> Product/3, Sum3/2
  Product/1 -> Mux1/3, Switch2/2, Switch1/2
  Sum2/1 -> Product/1
  Mux1/1 -> Scope2/1
  Relational Operator/1 -> Max. Reached?/1, Unit Delay1/1, Mux1/1
  Max. Num/1 -> Relational Operator/1
  Unit Delay/1 -> Switch1/1
  Sum/1 -> Mux1/2, Relational Operator/2, Unit Delay/1
  Switch2/1 -> Sum/2
  Switch1/1 -> Sum/1
  Constant3/1 -> Switch2/3
  Constant2/1 -> Switch2/1
  Constant1/1 -> Switch1/3

== system FOC_PMSM_FVSensorNew_testing/Rotor Pos. estimation/Cal. stator flux linkage1/MinMax detection/Min. Det/Counter.2/Conter with enable ==
  note: High input enables counting
      | Low input set the SR (output 1)
      | To be ready for next start of
      | counting
  note: Max. counter not reached - 0
      | reached, give a pulse, width
      | determined by the 1/z
  _|  |_ : Inport
  Max. Num : Inport  Port=2
  Constant1 : Constant  Value=0
  Constant2 : Constant
  Constant3 : Constant  Value=0
  Constant6 : Constant
  Constant7 : Constant
  Mux1 : Mux  Inputs=3
  Product : Product  Inputs=3  RndMeth=Zero
  Relational Operator : RelationalOperator  Operator=<=  RndMeth=Nearest
  SR Latch : Subsystem
  Scope2 : Scope
  Sum : Sum  Inputs=|++
  Sum2 : Sum  Inputs=-+|
  Sum3 : Sum  Inputs=+-|
  Switch1 : Switch  Threshold=0.5
  Switch2 : Switch  Threshold=0.5
  Unit Delay : UnitDelay  SampleTime=-1
  Unit Delay1 : UnitDelay  SampleTime=-1
  Max. Reached? : Outport
  wires:
  Constant1/1 -> Switch1/3
  Constant2/1 -> Switch2/1
  Constant3/1 -> Switch2/3
  Switch1/1 -> Sum/1
  Switch2/1 -> Sum/2
  Sum/1 -> Unit Delay/1, Relational Operator/2, Mux1/2
  Unit Delay/1 -> Switch1/1
  Max. Num/1 -> Relational Operator/1
  Relational Operator/1 -> Mux1/1, Unit Delay1/1, Max. Reached?/1
  Mux1/1 -> Scope2/1
  Sum2/1 -> Product/1
  Product/1 -> Switch1/2, Switch2/2, Mux1/3
  _|  |_/1 -> Sum3/2, Product/3
  SR Latch/1(Q) -> Product/2
  Sum3/1 -> SR Latch/2(S)
  Constant7/1 -> Sum3/1
  Constant6/1 -> Sum2/2
  Unit Delay1/1 -> Sum2/1, SR Latch/1(R)

== system FOC_PMSM_FVSensorNew_testing/Rotor Pos. estimation/Cal. stator flux linkage1/MinMax detection/Min. Det/Counter.2/Rising edge gen. ==
  note: Max. counter not reached - 0
      | reached, give a pulse, width
      | determined by the 1/z
  note: High input enables counting
      | Low input set the SR (output 1)
      | To be ready for next start of
      | counting
  _|  |_ : Inport
  Constant1 : Constant  Value=0
  Constant{2,4,6..7} (4 alike) : Constant
  Constant3 : Constant  Value=0
  Mux1 : Mux  Inputs=3
  Product : Product  Inputs=3  RndMeth=Zero
  Relational Operator : RelationalOperator  Operator=<=  RndMeth=Nearest
  SR Latch : Subsystem
  Scope2 : Scope
  Sum : Sum  Inputs=|++
  Sum2 : Sum  Inputs=-+|
  Sum3 : Sum  Inputs=+-|
  Switch1 : Switch  Threshold=0.5
  Switch2 : Switch  Threshold=0.5
  Unit Delay : UnitDelay  SampleTime=-1
  Unit Delay1 : UnitDelay  SampleTime=-1
  Edge : Outport
  wires:
  Unit Delay1/1 -> SR Latch/1(R), Sum2/1
  Constant6/1 -> Sum2/2
  Constant7/1 -> Sum3/1
  Sum3/1 -> SR Latch/2(S)
  SR Latch/1(Q) -> Product/2
  _|  |_/1 -> Product/3, Sum3/2
  Product/1 -> Mux1/3, Switch2/2, Switch1/2
  Sum2/1 -> Product/1
  Mux1/1 -> Scope2/1
  Relational Operator/1 -> Edge/1, Unit Delay1/1, Mux1/1
  Constant4/1 -> Relational Operator/1
  Unit Delay/1 -> Switch1/1
  Sum/1 -> Mux1/2, Relational Operator/2, Unit Delay/1
  Switch2/1 -> Sum/2
  Switch1/1 -> Sum/1
  Constant3/1 -> Switch2/3
  Constant2/1 -> Switch2/1
  Constant1/1 -> Switch1/3

== system FOC_PMSM_FVSensorNew_testing/Rotor Pos. estimation/Cal. stator flux linkage1/MinMax detection/Min. Det/Counter.2/SR Latch ==
  R : Inport
  S : Inport  Port=2
  Constant2 : Constant
  Constant4 : Constant  Value=0
  Constant5 : Constant  Value=0
  Multiport Switch : MultiPortSwitch  Inputs=4
  Mux1 : Mux  Inputs=2
  Selcect : Fcn  Expr=(1-u(1))*(1-u(2))+2*(1-u(1))*u(2)+3*u(1)*(1-u(2))+4*u(1)*u(2)
  Unit Delay2 : UnitDelay  SampleTime=-1
  Q : Outport
  wires:
  Multiport Switch/1 -> Q/1, Unit Delay2/1
  Selcect/1 -> Multiport Switch/1
  Mux1/1 -> Selcect/1
  Unit Delay2/1 -> Multiport Switch/2
  Constant2/1 -> Multiport Switch/3
  Constant4/1 -> Multiport Switch/4
  Constant5/1 -> Multiport Switch/5
  R/1 -> Mux1/1
  S/1 -> Mux1/2

== system FOC_PMSM_FVSensorNew_testing/Rotor Pos. estimation/Cal. stator flux linkage/MinMax detection/Max. Det/Counter.1/Conter with enable/SR Latch ==
  R : Inport
  S : Inport  Port=2
  Constant2 : Constant
  Constant4 : Constant  Value=0
  Constant5 : Constant  Value=0
  Multiport Switch : MultiPortSwitch  Inputs=4
  Mux1 : Mux  Inputs=2
  Selcect : Fcn  Expr=(1-u(1))*(1-u(2))+2*(1-u(1))*u(2)+3*u(1)*(1-u(2))+4*u(1)*u(2)
  Unit Delay2 : UnitDelay  SampleTime=-1
  Q : Outport
  wires:
  Multiport Switch/1 -> Q/1, Unit Delay2/1
  Selcect/1 -> Multiport Switch/1
  Mux1/1 -> Selcect/1
  Unit Delay2/1 -> Multiport Switch/2
  Constant2/1 -> Multiport Switch/3
  Constant4/1 -> Multiport Switch/4
  Constant5/1 -> Multiport Switch/5
  R/1 -> Mux1/1
  S/1 -> Mux1/2

== system FOC_PMSM_FVSensorNew_testing/Rotor Pos. estimation/Cal. stator flux linkage/MinMax detection/Max. Det/Counter.2/Conter with enable/SR Latch ==
  R : Inport
  S : Inport  Port=2
  Constant2 : Constant
  Constant4 : Constant  Value=0
  Constant5 : Constant  Value=0
  Multiport Switch : MultiPortSwitch  Inputs=4
  Mux1 : Mux  Inputs=2
  Selcect : Fcn  Expr=(1-u(1))*(1-u(2))+2*(1-u(1))*u(2)+3*u(1)*(1-u(2))+4*u(1)*u(2)
  Unit Delay2 : UnitDelay  SampleTime=-1
  Q : Outport
  wires:
  S/1 -> Mux1/2
  R/1 -> Mux1/1
  Constant5/1 -> Multiport Switch/5
  Constant4/1 -> Multiport Switch/4
  Constant2/1 -> Multiport Switch/3
  Unit Delay2/1 -> Multiport Switch/2
  Mux1/1 -> Selcect/1
  Selcect/1 -> Multiport Switch/1
  Multiport Switch/1 -> Unit Delay2/1, Q/1

== system FOC_PMSM_FVSensorNew_testing/Rotor Pos. estimation/Cal. stator flux linkage/MinMax detection/Max. Det/Counter.2/Rising edge gen./SR Latch ==
  R : Inport
  S : Inport  Port=2
  Constant2 : Constant
  Constant4 : Constant  Value=0
  Constant5 : Constant  Value=0
  Multiport Switch : MultiPortSwitch  Inputs=4
  Mux1 : Mux  Inputs=2
  Selcect : Fcn  Expr=(1-u(1))*(1-u(2))+2*(1-u(1))*u(2)+3*u(1)*(1-u(2))+4*u(1)*u(2)
  Unit Delay2 : UnitDelay  SampleTime=-1
  Q : Outport
  wires:
  Multiport Switch/1 -> Q/1, Unit Delay2/1
  Selcect/1 -> Multiport Switch/1
  Mux1/1 -> Selcect/1
  Unit Delay2/1 -> Multiport Switch/2
  Constant2/1 -> Multiport Switch/3
  Constant4/1 -> Multiport Switch/4
  Constant5/1 -> Multiport Switch/5
  R/1 -> Mux1/1
  S/1 -> Mux1/2

== system FOC_PMSM_FVSensorNew_testing/Rotor Pos. estimation/Cal. stator flux linkage/MinMax detection/Min. Det/Counter.1/Conter with enable/SR Latch ==
  R : Inport
  S : Inport  Port=2
  Constant2 : Constant
  Constant4 : Constant  Value=0
  Constant5 : Constant  Value=0
  Multiport Switch : MultiPortSwitch  Inputs=4
  Mux1 : Mux  Inputs=2
  Selcect : Fcn  Expr=(1-u(1))*(1-u(2))+2*(1-u(1))*u(2)+3*u(1)*(1-u(2))+4*u(1)*u(2)
  Unit Delay2 : UnitDelay  SampleTime=-1
  Q : Outport
  wires:
  S/1 -> Mux1/2
  R/1 -> Mux1/1
  Constant5/1 -> Multiport Switch/5
  Constant4/1 -> Multiport Switch/4
  Constant2/1 -> Multiport Switch/3
  Unit Delay2/1 -> Multiport Switch/2
  Mux1/1 -> Selcect/1
  Selcect/1 -> Multiport Switch/1
  Multiport Switch/1 -> Unit Delay2/1, Q/1

== system FOC_PMSM_FVSensorNew_testing/Rotor Pos. estimation/Cal. stator flux linkage/MinMax detection/Min. Det/Counter.2/Conter with enable/SR Latch ==
  R : Inport
  S : Inport  Port=2
  Constant2 : Constant
  Constant4 : Constant  Value=0
  Constant5 : Constant  Value=0
  Multiport Switch : MultiPortSwitch  Inputs=4
  Mux1 : Mux  Inputs=2
  Selcect : Fcn  Expr=(1-u(1))*(1-u(2))+2*(1-u(1))*u(2)+3*u(1)*(1-u(2))+4*u(1)*u(2)
  Unit Delay2 : UnitDelay  SampleTime=-1
  Q : Outport
  wires:
  Multiport Switch/1 -> Q/1, Unit Delay2/1
  Selcect/1 -> Multiport Switch/1
  Mux1/1 -> Selcect/1
  Unit Delay2/1 -> Multiport Switch/2
  Constant2/1 -> Multiport Switch/3
  Constant4/1 -> Multiport Switch/4
  Constant5/1 -> Multiport Switch/5
  R/1 -> Mux1/1
  S/1 -> Mux1/2

== system FOC_PMSM_FVSensorNew_testing/Rotor Pos. estimation/Cal. stator flux linkage/MinMax detection/Min. Det/Counter.2/Rising edge gen./SR Latch ==
  R : Inport
  S : Inport  Port=2
  Constant2 : Constant
  Constant4 : Constant  Value=0
  Constant5 : Constant  Value=0
  Multiport Switch : MultiPortSwitch  Inputs=4
  Mux1 : Mux  Inputs=2
  Selcect : Fcn  Expr=(1-u(1))*(1-u(2))+2*(1-u(1))*u(2)+3*u(1)*(1-u(2))+4*u(1)*u(2)
  Unit Delay2 : UnitDelay  SampleTime=-1
  Q : Outport
  wires:
  S/1 -> Mux1/2
  R/1 -> Mux1/1
  Constant5/1 -> Multiport Switch/5
  Constant4/1 -> Multiport Switch/4
  Constant2/1 -> Multiport Switch/3
  Unit Delay2/1 -> Multiport Switch/2
  Mux1/1 -> Selcect/1
  Selcect/1 -> Multiport Switch/1
  Multiport Switch/1 -> Unit Delay2/1, Q/1

== system FOC_PMSM_FVSensorNew_testing/Rotor Pos. estimation/Cal. stator flux linkage1/MinMax detection/Max. Det/Counter.1/Conter with enable/SR Latch ==
  R : Inport
  S : Inport  Port=2
  Constant2 : Constant
  Constant4 : Constant  Value=0
  Constant5 : Constant  Value=0
  Multiport Switch : MultiPortSwitch  Inputs=4
  Mux1 : Mux  Inputs=2
  Selcect : Fcn  Expr=(1-u(1))*(1-u(2))+2*(1-u(1))*u(2)+3*u(1)*(1-u(2))+4*u(1)*u(2)
  Unit Delay2 : UnitDelay  SampleTime=-1
  Q : Outport
  wires:
  Multiport Switch/1 -> Q/1, Unit Delay2/1
  Selcect/1 -> Multiport Switch/1
  Mux1/1 -> Selcect/1
  Unit Delay2/1 -> Multiport Switch/2
  Constant2/1 -> Multiport Switch/3
  Constant4/1 -> Multiport Switch/4
  Constant5/1 -> Multiport Switch/5
  R/1 -> Mux1/1
  S/1 -> Mux1/2

== system FOC_PMSM_FVSensorNew_testing/Rotor Pos. estimation/Cal. stator flux linkage1/MinMax detection/Max. Det/Counter.2/Conter with enable/SR Latch ==
  R : Inport
  S : Inport  Port=2
  Constant2 : Constant
  Constant4 : Constant  Value=0
  Constant5 : Constant  Value=0
  Multiport Switch : MultiPortSwitch  Inputs=4
  Mux1 : Mux  Inputs=2
  Selcect : Fcn  Expr=(1-u(1))*(1-u(2))+2*(1-u(1))*u(2)+3*u(1)*(1-u(2))+4*u(1)*u(2)
  Unit Delay2 : UnitDelay  SampleTime=-1
  Q : Outport
  wires:
  S/1 -> Mux1/2
  R/1 -> Mux1/1
  Constant5/1 -> Multiport Switch/5
  Constant4/1 -> Multiport Switch/4
  Constant2/1 -> Multiport Switch/3
  Unit Delay2/1 -> Multiport Switch/2
  Mux1/1 -> Selcect/1
  Selcect/1 -> Multiport Switch/1
  Multiport Switch/1 -> Unit Delay2/1, Q/1

== system FOC_PMSM_FVSensorNew_testing/Rotor Pos. estimation/Cal. stator flux linkage1/MinMax detection/Max. Det/Counter.2/Rising edge gen./SR Latch ==
  R : Inport
  S : Inport  Port=2
  Constant2 : Constant
  Constant4 : Constant  Value=0
  Constant5 : Constant  Value=0
  Multiport Switch : MultiPortSwitch  Inputs=4
  Mux1 : Mux  Inputs=2
  Selcect : Fcn  Expr=(1-u(1))*(1-u(2))+2*(1-u(1))*u(2)+3*u(1)*(1-u(2))+4*u(1)*u(2)
  Unit Delay2 : UnitDelay  SampleTime=-1
  Q : Outport
  wires:
  Multiport Switch/1 -> Q/1, Unit Delay2/1
  Selcect/1 -> Multiport Switch/1
  Mux1/1 -> Selcect/1
  Unit Delay2/1 -> Multiport Switch/2
  Constant2/1 -> Multiport Switch/3
  Constant4/1 -> Multiport Switch/4
  Constant5/1 -> Multiport Switch/5
  R/1 -> Mux1/1
  S/1 -> Mux1/2

== system FOC_PMSM_FVSensorNew_testing/Rotor Pos. estimation/Cal. stator flux linkage1/MinMax detection/Min. Det/Counter.1/Conter with enable/SR Latch ==
  R : Inport
  S : Inport  Port=2
  Constant2 : Constant
  Constant4 : Constant  Value=0
  Constant5 : Constant  Value=0
  Multiport Switch : MultiPortSwitch  Inputs=4
  Mux1 : Mux  Inputs=2
  Selcect : Fcn  Expr=(1-u(1))*(1-u(2))+2*(1-u(1))*u(2)+3*u(1)*(1-u(2))+4*u(1)*u(2)
  Unit Delay2 : UnitDelay  SampleTime=-1
  Q : Outport
  wires:
  S/1 -> Mux1/2
  R/1 -> Mux1/1
  Constant5/1 -> Multiport Switch/5
  Constant4/1 -> Multiport Switch/4
  Constant2/1 -> Multiport Switch/3
  Unit Delay2/1 -> Multiport Switch/2
  Mux1/1 -> Selcect/1
  Selcect/1 -> Multiport Switch/1
  Multiport Switch/1 -> Unit Delay2/1, Q/1

== system FOC_PMSM_FVSensorNew_testing/Rotor Pos. estimation/Cal. stator flux linkage1/MinMax detection/Min. Det/Counter.2/Conter with enable/SR Latch ==
  R : Inport
  S : Inport  Port=2
  Constant2 : Constant
  Constant4 : Constant  Value=0
  Constant5 : Constant  Value=0
  Multiport Switch : MultiPortSwitch  Inputs=4
  Mux1 : Mux  Inputs=2
  Selcect : Fcn  Expr=(1-u(1))*(1-u(2))+2*(1-u(1))*u(2)+3*u(1)*(1-u(2))+4*u(1)*u(2)
  Unit Delay2 : UnitDelay  SampleTime=-1
  Q : Outport
  wires:
  Multiport Switch/1 -> Q/1, Unit Delay2/1
  Selcect/1 -> Multiport Switch/1
  Mux1/1 -> Selcect/1
  Unit Delay2/1 -> Multiport Switch/2
  Constant2/1 -> Multiport Switch/3
  Constant4/1 -> Multiport Switch/4
  Constant5/1 -> Multiport Switch/5
  R/1 -> Mux1/1
  S/1 -> Mux1/2

== system FOC_PMSM_FVSensorNew_testing/Rotor Pos. estimation/Cal. stator flux linkage1/MinMax detection/Min. Det/Counter.2/Rising edge gen./SR Latch ==
  R : Inport
  S : Inport  Port=2
  Constant2 : Constant
  Constant4 : Constant  Value=0
  Constant5 : Constant  Value=0
  Multiport Switch : MultiPortSwitch  Inputs=4
  Mux1 : Mux  Inputs=2
  Selcect : Fcn  Expr=(1-u(1))*(1-u(2))+2*(1-u(1))*u(2)+3*u(1)*(1-u(2))+4*u(1)*u(2)
  Unit Delay2 : UnitDelay  SampleTime=-1
  Q : Outport
  wires:
  S/1 -> Mux1/2
  R/1 -> Mux1/1
  Constant5/1 -> Multiport Switch/5
  Constant4/1 -> Multiport Switch/4
  Constant2/1 -> Multiport Switch/3
  Unit Delay2/1 -> Multiport Switch/2
  Mux1/1 -> Selcect/1
  Selcect/1 -> Multiport Switch/1
  Multiport Switch/1 -> Unit Delay2/1, Q/1
